simulink library "pathGeometryEn_ul"  (R2020a)
settings: Solver=VariableStepAuto  StartTime=0.0  StopTime=10.0  RelTol=1e-3
settings Model: Creator=mcobb  LastModifiedBy=JohnJr
settings DataIOCC: ReturnWorkspaceOutputs=off
settings DebuggingCC: ArithmeticOperatorsInVariantConditions=warning
settings SFSimCC: CustomCodeUndefinedFunction=UseInterfaceOnly

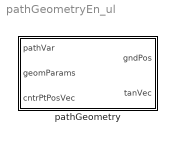
== system pathGeometryEn_ul ==
  pathGeometry : Subsystem

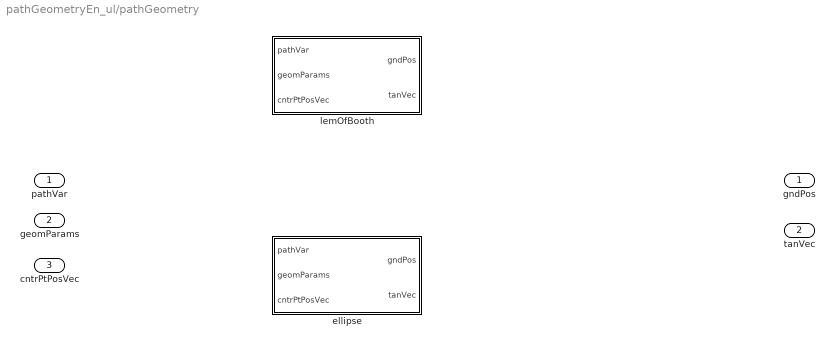
== system pathGeometryEn_ul/pathGeometry ==
  pathVar : Inport
  geomParams : Inport  Port=2
  cntrPtPosVec : Inport  Port=3
  ellipse : Subsystem
  lemOfBooth : Subsystem
  gndPos : Outport
  tanVec : Outport  Port=2

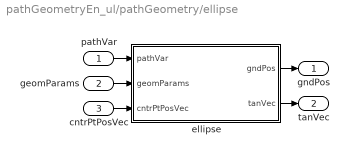
== system pathGeometryEn_ul/pathGeometry/ellipse ==
  pathVar : Inport
  geomParams : Inport  Port=2
  cntrPtPosVec : Inport  Port=3
  ellipse : MATLAB Function  TreatAsAtomicUnit=on  VariantControl=VSS_pathGeometry_ellipse
  gndPos : Outport
  tanVec : Outport  Port=2
  wires:
  ellipse/2(tanVec) -> tanVec/1
  geomParams/1 -> ellipse/2(geomParams)
  cntrPtPosVec/1 -> ellipse/3(cntrPtPosVec)
  ellipse/1(gndPos) -> gndPos/1
  pathVar/1 -> ellipse/1(pathVar)

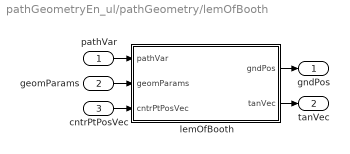
== system pathGeometryEn_ul/pathGeometry/lemOfBooth ==
  pathVar : Inport
  geomParams : Inport  Port=2
  cntrPtPosVec : Inport  Port=3
  lemOfBooth : MATLAB Function  TreatAsAtomicUnit=on  VariantControl=VSS_pathGeometry_lemOfBooth
  gndPos : Outport
  tanVec : Outport  Port=2
  wires:
  geomParams/1 -> lemOfBooth/2(geomParams)
  pathVar/1 -> lemOfBooth/1(pathVar)
  cntrPtPosVec/1 -> lemOfBooth/3(cntrPtPosVec)
  lemOfBooth/1(gndPos) -> gndPos/1
  lemOfBooth/2(tanVec) -> tanVec/1

== matlab function pathGeometryEn_ul/pathGeometry/ellipse/ellipse ==
  data: pathVar input; gndPos output; geomParams input; tanVec output; cntrPtPosVec input
function [gndPos,tanVec] = fcn(pathVar,geomParams,cntrPtPosVec)
[gndPos,tanVec] = ellipse(pathVar,geomParams,cntrPtPosVec);

== matlab function pathGeometryEn_ul/pathGeometry/lemOfBooth/lemOfBooth ==
  data: pathVar input; gndPos output; geomParams input; tanVec output; cntrPtPosVec input
function [gndPos,tanVec] = fcn(pathVar,geomParams,cntrPtPosVec)
[gndPos,tanVec] = lemOfBooth(pathVar,geomParams,cntrPtPosVec);
